simulink model "MSD_simulink"  (R2023b)
settings: Solver=VariableStepAuto  StartTime=0.0  StopTime=Tf  RelTol=1e-3
values from neighbouring files (symbols this model uses):
  A = [-r/m, -k/m; 1, 0]    [Mass_spring_damper_main.m]
  B = [1/m; 0]    [Mass_spring_damper_main.m]
  C = eye(2)    [Mass_spring_damper_main.m]
  D = zeros(2,1)    [Mass_spring_damper_main.m]    (also in project.m = tf(numD, denD); project_section_1.m = tf(num_D,den_D))
  k = 1    [Mass_spring_damper_main.m]    (also in PD_main.m; asymp.m = numdeg+1; second_exercise_exam_example.m)
  Kp = 100    [Mass_spring_damper_main.m]    (also in project.m = 5)
  m = 1    [Mass_spring_damper_main.m]    (also in PD_main.m; project_2dof.m = 1500)
  r = 10    [Mass_spring_damper_main.m]    (also in second_exercise_exam_example.m = -1)
  x_ref = 1    [Mass_spring_damper_main.m]
settings Model: Creator=emanu  LastModifiedBy=fra12
settings SolverCC: AlgebraicLoopSolver=TrustRegion
settings DebuggingCC: UnconnectedInputMsg=warning  UnconnectedOutputMsg=warning  UnconnectedLineMsg=warning
settings ModelReferenceCC: EnableRefExpFcnMdlSchedulingChecks=on

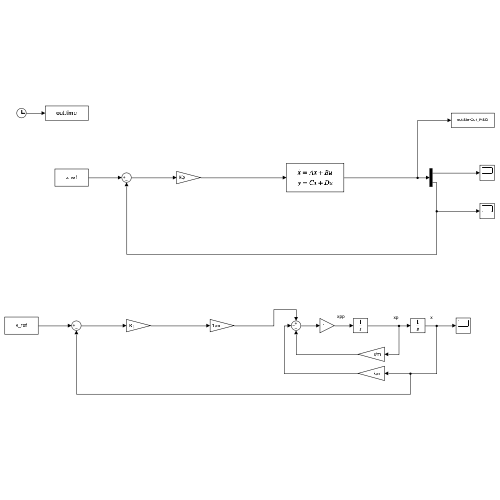
[thumbnail: Simulink's stored preview of the top-level diagram]
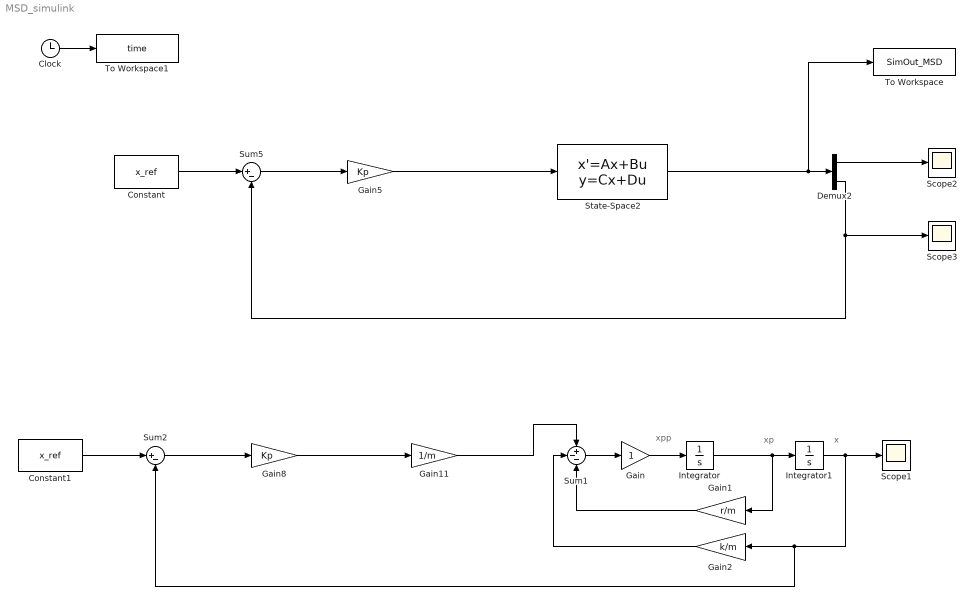
== system MSD_simulink ==
  note: x
  note: xp
  note: xpp
  Clock : Clock
  Constant : Constant  Value=x_ref
  Constant1 : Constant  Value=x_ref
  Demux2 : Demux  Outputs=2
  Gain : Gain
  Gain1 : Gain  Gain=r/m
  Gain11 : Gain  Gain=1/m
  Gain2 : Gain  Gain=k/m
  Gain5 : Gain  Gain=Kp
  Gain8 : Gain  Gain=Kp
  Integrator : Integrator
  Integrator1 : Integrator
  Scope1 : Scope
  Scope2 : Scope
  Scope3 : Scope
  State-Space2 : StateSpace  A=A  B=B  C=C  D=D  InitialCondition=0
  Sum1 : Sum  Inputs=+--
  Sum2 : Sum  Inputs=|+-
  Sum5 : Sum  Inputs=|+-
  To Workspace : ToWorkspace  VariableName=SimOut_MSD  SampleTime=-1
  To Workspace1 : ToWorkspace  VariableName=time  SaveFormat=Timeseries  SampleTime=-1
  wires:
  Gain/1 -> Integrator/1
  Integrator/1 -> Gain1/1, Integrator1/1
  Gain1/1 -> Sum1/3
  Integrator1/1 -> Gain2/1, Sum2/2, Scope1/1
  Gain2/1 -> Sum1/2
  Sum1/1 -> Gain/1
  Clock/1 -> To Workspace1/1
  Demux2/2 -> Scope3/1, Sum5/2
  State-Space2/1 -> To Workspace/1, Demux2/1
  Sum5/1 -> Gain5/1
  Constant/1 -> Sum5/1
  Constant1/1 -> Sum2/1
  Sum2/1 -> Gain8/1
  Gain5/1 -> State-Space2/1
  Gain11/1 -> Sum1/1
  Gain8/1 -> Gain11/1
  Demux2/1 -> Scope2/1
